simulink model "corripd1"  (Simulink 5.0)
settings: Solver=ode45  StartTime=0.0  StopTime=2.335  MaxStep=0.001  MinStep=0.001  RelTol=1e-3  AbsTol=1e-3
values from neighbouring files (symbols this model uses):
  b = 5E-5    (= 5e-05)    [Constants.m]
  J = 1    [Constants.m]
  Ka = 20    [Constants.m]
  Km = 1.36    [Constants.m]
  Kp = 50    [Constants.m]
  Kv = Kvc    [Constants.m]
  tm = 0.001    [Constants.m]
settings Model: LastModifiedBy=rzotovic  SaveTime=off  SaveOutput=off

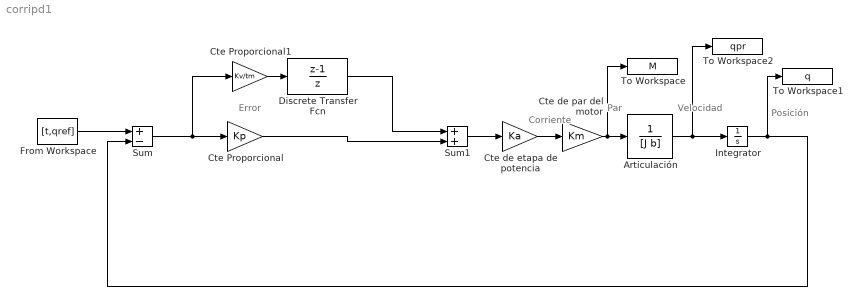
== system corripd1 ==
  note: Corriente
  note: Error
  note: Par
  note: Velocidad
  note: Posición
  Articulación : TransferFcn  Denominator=[J b]
  Cte Proporcional : Gain  Gain=Kp  SaturateOnIntegerOverflow=on
  Cte Proporcional1 : Gain  Gain=Kv/tm  SaturateOnIntegerOverflow=on
  Cte de etapa de potencia : Gain  Gain=Ka  SaturateOnIntegerOverflow=on
  Cte de par del motor : Gain  Gain=Km  SaturateOnIntegerOverflow=on
  Discrete Transfer Fcn : DiscreteTransferFcn  Numerator=[1 -1]  Denominator=[1 0]  SampleTime=tm
  From Workspace : FromWorkspace  VariableName=[t,qref]
  Integrator : Integrator
  Sum : Sum  Inputs=+-  SaturateOnIntegerOverflow=on  InputSameDT=on
  Sum1 : Sum  SaturateOnIntegerOverflow=on  InputSameDT=on
  To Workspace : ToWorkspace  VariableName=M  SaveFormat=Array
      settings: MaxDataPoints=2335
  To Workspace1 : ToWorkspace  VariableName=q  SaveFormat=Array
      settings: MaxDataPoints=2335
  To Workspace2 : ToWorkspace  VariableName=qpr  SaveFormat=Array
      settings: MaxDataPoints=2335
  wires:
  Cte de par del motor/1 -> Articulación/1, To Workspace/1
  Articulación/1 -> Integrator/1, To Workspace2/1
  Cte de etapa de potencia/1 -> Cte de par del motor/1
  From Workspace/1 -> Sum/1
  Sum/1 -> Cte Proporcional/1, Cte Proporcional1/1
  Integrator/1 -> Sum/2, To Workspace1/1
  Sum1/1 -> Cte de etapa de potencia/1
  Cte Proporcional1/1 -> Discrete Transfer Fcn/1
  Discrete Transfer Fcn/1 -> Sum1/1
  Cte Proporcional/1 -> Sum1/2
